simulink model "susp_utf8"  (Simulink 8.1)
settings: Solver=ode45  StartTime=0.0  StopTime=5  RelTol=1e-6
values from neighbouring files (symbols this model uses):
  A = [0 1 0 0;-(kf/ms) -(ba/ms) (kf/ms) (ba/ms); 0 0 0 1; (kf/mr) (ba/mr) -(kf+kp)/mr -(ba/mr)]    [dados_susp.m]
  B = [0 0;0 -1/ms; 0 0;(kp/mr) (1/mr)]    [dados_susp.m]
  C = [1 0 0 0;0 1 0 0;0 0 1 0;0 0 0 1]    [dados_susp.m]
  Coff = 500    [dados_susp.m]
  Con = 1400    [dados_susp.m]
  D = [0 0; 0 0; 0 0; 0 0]    [dados_susp.m]
undefined symbols (not defined in the file or in its folder): SEL
libraries: fuzblock x2
settings Model: Creator=dello  LastModifiedBy=dello
settings DataIOCC: SignalLoggingName=sigsOut
settings OptimizationCC: ExpressionDepthLimit=128  InitFltsAndDblsToZero=on
settings DebuggingCC: SaveWithParameterizedLinksMsg=none  SignalResolutionControl=TryResolveAllWithWarning  SolverPrmCheckMsg=none  MultiTaskDSMMsg=warning  MultiTaskCondExecSysMsg=none  StrictBusMsg=None
settings HardwareCC: TargetUnknown=on
settings RTWCC: IncludeERTFirstTime=on
settings GRTTargetCC: TargetFcnLib=ansi_tfl_tmw.mat

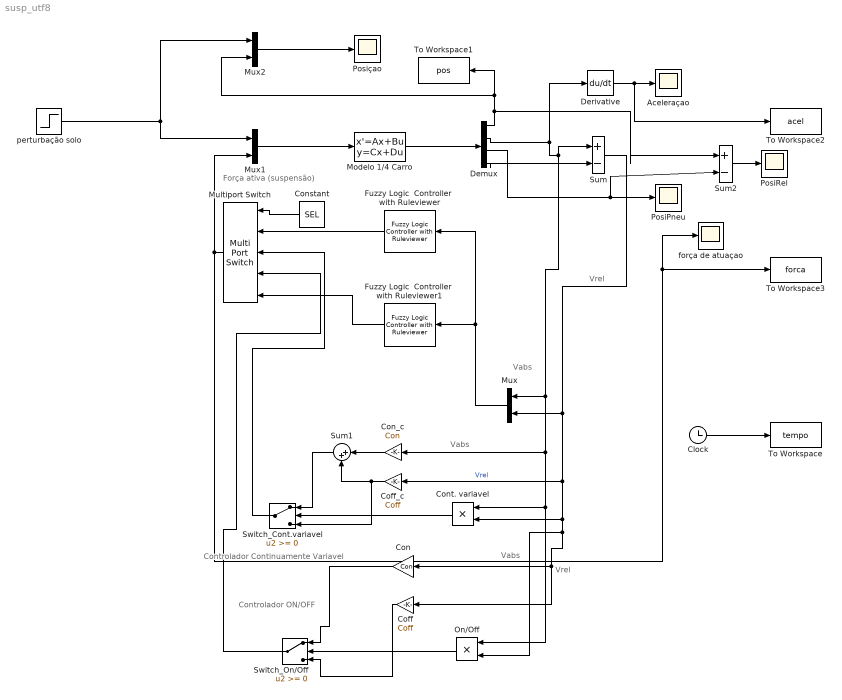
== system susp_utf8 ==
  note: Vrel
  note: Vabs
  note: Vabs
  note: Vabs
  note: Vrel
  note: Força ativa (suspensão)
  note: Controlador
      | Continuamente Variavel
  note: Controlador ON/OFF
  Aceleraçao : Scope
      settings: TimeRange=2  YMin=-9  SaveName=Aceleracao
  Clock : Clock
  Coff : Gain  Gain=Coff  SaturateOnIntegerOverflow=on  OutDataTypeStr=Inherit: Same as input  ParamDataTypeStr=Inherit: Same as input
  Coff_c : Gain  Gain=Coff  SaturateOnIntegerOverflow=on  OutDataTypeStr=Inherit: Same as input  ParamDataTypeStr=Inherit: Same as input
  Con : Gain  Gain=Con  SaturateOnIntegerOverflow=on  OutDataTypeStr=Inherit: Same as input  ParamDataTypeStr=Inherit: Same as input
  Con_c : Gain  Gain=Con  SaturateOnIntegerOverflow=on  OutDataTypeStr=Inherit: Same as input  ParamDataTypeStr=Inherit: Same as input
  Constant : Constant  Value=SEL
  Cont. variavel : Product  SaturateOnIntegerOverflow=on  OutDataTypeStr=Inherit: Same as first input
  Demux : Demux
  Derivative : Derivative
  Fuzzy Logic  Controller  with Ruleviewer : fuzblock/Fuzzy Logic  Controller  with Ruleviewer  fismatrix=fis2  Ts=2
  Fuzzy Logic  Controller  with Ruleviewer1 : fuzblock/Fuzzy Logic  Controller  with Ruleviewer  fismatrix=fis3  Ts=2
  Modelo 1/4 Carro : StateSpace  A=A  B=B  C=C  D=D  X0=[0 0 0 0]
  Multiport Switch : MultiPortSwitch  Inputs=4
  Mux : Mux  Inputs=2
  Mux1 : Mux  Inputs=2
  Mux2 : Mux  Inputs=2
  On/Off : Product  SaturateOnIntegerOverflow=on  OutDataTypeStr=Inherit: Same as first input
  PosiPneu : Scope
      settings: TimeRange=2  YMin=0.0375  YMax=0.0875  SaveName=posicao_chassis1
  PosiRel : Scope
      settings: TimeRange=2  YMin=-0.17  YMax=0.01  SaveName=posicao_chassis2
  Posiçao : Scope
      settings: TimeRange=1  YMin=0.036  YMax=0.05  SaveName=posicao_chassis
  Sum : Sum  Inputs=|+-  SaturateOnIntegerOverflow=on
  Sum1 : Sum  Inputs=|++  SaturateOnIntegerOverflow=on
  Sum2 : Sum  Inputs=|+-  SaturateOnIntegerOverflow=on
  Switch_Cont.variavel : Switch  SaturateOnIntegerOverflow=on
  Switch_On/Off : Switch  SaturateOnIntegerOverflow=on
  To Workspace : ToWorkspace  VariableName=tempo  SampleTime=-1
  To Workspace1 : ToWorkspace  VariableName=pos  SampleTime=-1
  To Workspace2 : ToWorkspace  VariableName=acel  SampleTime=-1
  To Workspace3 : ToWorkspace  VariableName=forca  SampleTime=-1
  força de atuaçao : Scope
      settings: TimeRange=2  YMin=-2  YMax=1  SaveName=Aceleraao1
  perturbação solo : Step  Time=0  After=0.05  SampleTime=0  VectorParams1D=off  ZeroCross=off
  wires:
  Modelo 1/4 Carro/1 -> Demux/1
  Mux1/1 -> Modelo 1/4 Carro/1
  Demux/4 -> Sum/2
  Demux/2 -> Sum/1, On/Off/1, Cont. variavel/1, Con_c/1, Mux/1, Derivative/1
  Derivative/1 -> Aceleraçao/1, To Workspace2/1
  Demux/1 -> Sum2/1, To Workspace1/1, Mux2/2
  Sum/1 -> Mux/2, Coff/1, Con/1, On/Off/2, Cont. variavel/2, Coff_c/1  "Vrel"
  Cont. variavel/1 -> Switch_Cont.variavel/2
  Coff_c/1 -> Sum1/2, Switch_Cont.variavel/3
  Con_c/1 -> Sum1/1
  Sum1/1 -> Switch_Cont.variavel/1
  Clock/1 -> To Workspace/1
  On/Off/1 -> Switch_On/Off/2
  Con/1 -> Switch_On/Off/1
  Coff/1 -> Switch_On/Off/3
  Mux/1 -> Fuzzy Logic  Controller  with Ruleviewer1/1, Fuzzy Logic  Controller  with Ruleviewer/1
  Demux/3 -> Sum2/2, PosiPneu/1
  Sum2/1 -> PosiRel/1
  Fuzzy Logic  Controller  with Ruleviewer/1 -> Multiport Switch/2
  Multiport Switch/1 -> To Workspace3/1, força de atuaçao/1, Mux1/2
  Mux2/1 -> Posiçao/1
  Switch_Cont.variavel/1 -> Multiport Switch/3
  Switch_On/Off/1 -> Multiport Switch/4
  perturbação solo/1 -> Mux1/1, Mux2/1
  Constant/1 -> Multiport Switch/1
  Fuzzy Logic  Controller  with Ruleviewer1/1 -> Multiport Switch/5
